simulink model "simulink_test1slx"  (R2022a)
settings: Solver=FixedStepAuto  StartTime=0.0  StopTime=50  FixedStep=0.01  RelTol=1e-3
libraries: simulink x2
settings Model: Creator=LENOVO  LastModifiedBy=LENOVO
settings DataIOCC: InspectSignalLogs=on

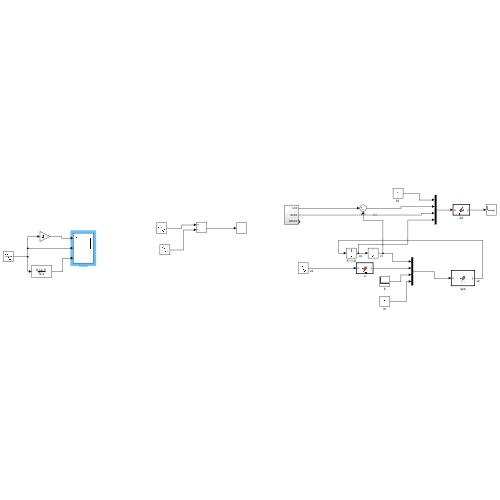
[thumbnail: Simulink's stored preview of the top-level diagram]
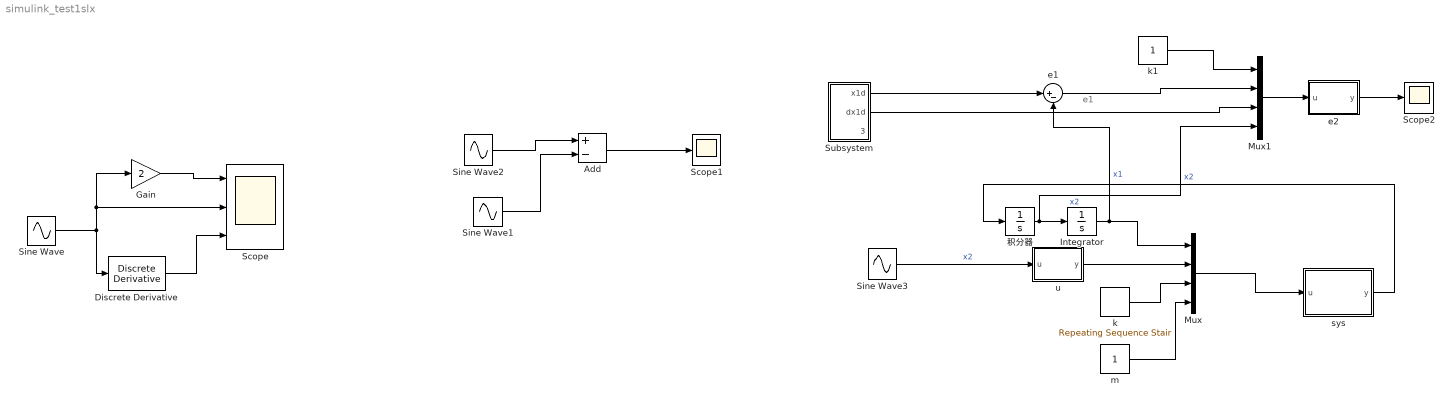
== system simulink_test1slx ==
  note: e1
  Add : Sum  Inputs=+-
  Discrete Derivative : simulink/Discrete/Discrete Derivative  gainval=1.0  ICPrevScaledInput=0.0  OutMin=[]  OutMax=[]  OutDataType=fixdt(1, 16)  OutScaling=2^-10  DoSatur=off
  Gain : Gain  Gain=2
  Integrator : Integrator
  Mux : Mux
  Mux1 : Mux
  Scope : Scope  NumInputPorts=3
  Scope1 : Scope
  Scope2 : Scope
  Sine Wave : Sin  SampleTime=0
  Sine Wave1 : Sin  Frequency=2  SampleTime=0
  Sine Wave2 : Sin  SampleTime=0
  Sine Wave3 : Sin  SampleTime=0
  Subsystem : Subsystem
  e1 : Sum  Inputs=|+-
  e2 : MATLAB Function  TreatAsAtomicUnit=on
  k : simulink/Sources/Repeating Sequence Stair  OutValues=[8].'  tsamp=25  OutMin=[]  OutMax=[]  OutDataTypeStr=double  OutputDataTypeScalingMode=double  OutDataType=fixdt(0,8)  ConRadixGroup=Best Precision: Vector-wise  OutScaling=2^-12
  k1 : Constant
  m : Constant
  sys : MATLAB Function  TreatAsAtomicUnit=on
  u : MATLAB Function  TreatAsAtomicUnit=on
  积分器 : Integrator
  wires:
  Sine Wave/1 -> Scope/2, Gain/1, Discrete Derivative/1
  Gain/1 -> Scope/1
  Discrete Derivative/1 -> Scope/3
  Sine Wave2/1 -> Add/1
  Sine Wave1/1 -> Add/2
  Add/1 -> Scope1/1
  积分器/1 -> Integrator/1, Mux1/4  "x2"
  Integrator/1 -> Mux/1, e1/2  "x1"
  Mux/1 -> sys/1(u)
  k/1 -> Mux/3
  m/1 -> Mux/4
  u/1(y) -> Mux/2
  sys/1(y) -> 积分器/1  "x2"
  Subsystem/1(x1d) -> e1/1
  Subsystem/2(dx1d) -> Mux1/3
  e1/1 -> Mux1/2
  k1/1 -> Mux1/1
  Mux1/1 -> e2/1(u)
  e2/1(y) -> Scope2/1
  Sine Wave3/1 -> u/1(u)  "x2"

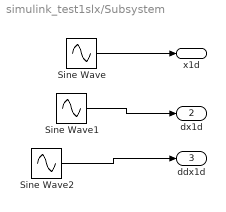
== system simulink_test1slx/Subsystem ==
  Sine Wave : Sin  SampleTime=0
  Sine Wave1 : Sin  SampleTime=0
  Sine Wave2 : Sin  SampleTime=0
  x1d : Outport
  dx1d : Outport  Port=2
  ddx1d : Outport  Port=3
  wires:
  Sine Wave/1 -> x1d/1
  Sine Wave1/1 -> dx1d/1
  Sine Wave2/1 -> ddx1d/1

== matlab function simulink_test1slx/sys ==
  data: u input; y output
function y = fcn(u)

y = -u(3)/u(4)*u(1)^3+1/u(4)*u(2);

== matlab function simulink_test1slx/e2 ==
  data: u input; y output
function y = fcn(u)

y = u(3)+u(1)*u(2)-(4);

== matlab function simulink_test1slx/u ==
  data: u input; y output
function y = fcn(u)

y = u;
